simulink model "engine_control_main_sim"  (R2022b)
settings: Solver=VariableStepAuto  StartTime=0.0  StopTime=10.0  RelTol=1e-3
libraries: cstblocks x8
settings Model: Creator=phatdo  LastModifiedBy=phatdo
settings DataIOCC: ReturnWorkspaceOutputs=off

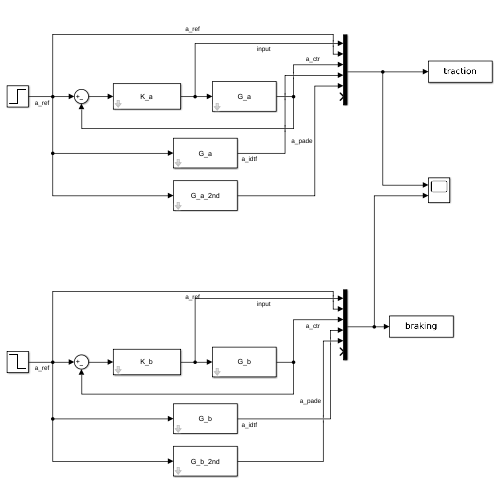
[thumbnail: Simulink's stored preview of the top-level diagram]
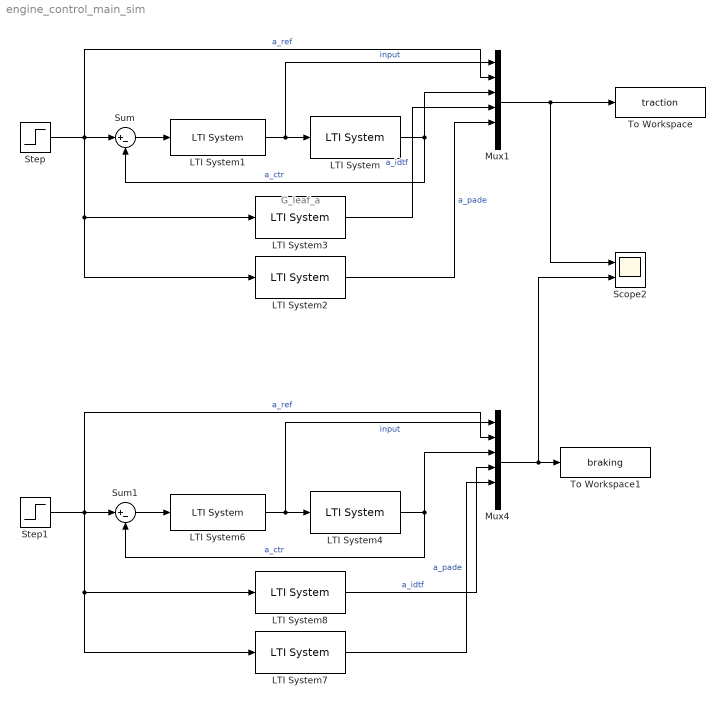
== system engine_control_main_sim ==
  note: G_leaf_a
  LTI System : cstblocks/LTI System  sys=G_a  IC=[]
  LTI System1 : cstblocks/LTI System  sys=K_a  IC=[]
  LTI System2 : cstblocks/LTI System  sys=G_a_2nd  IC=[]
  LTI System3 : cstblocks/LTI System  sys=G_a  IC=[]
  LTI System4 : cstblocks/LTI System  sys=G_b  IC=[]
  LTI System6 : cstblocks/LTI System  sys=K_b  IC=[]
  LTI System7 : cstblocks/LTI System  sys=G_b_2nd  IC=[]
  LTI System8 : cstblocks/LTI System  sys=G_b  IC=[]
  Mux1 : Mux  Inputs=6
  Mux4 : Mux  Inputs=6
  Scope2 : Scope  NumInputPorts=2
  Step : Step  SampleTime=0
  Step1 : Step  After=-1  SampleTime=0
  Sum : Sum  Inputs=|+-
  Sum1 : Sum  Inputs=|+-
  To Workspace : ToWorkspace  VariableName=traction  SaveFormat=Timeseries  SampleTime=-1
  To Workspace1 : ToWorkspace  VariableName=braking  SaveFormat=Timeseries  SampleTime=-1
  wires:
  Step/1 -> Mux1/2, LTI System3/1, LTI System2/1, Sum/1  "a_ref"
  LTI System1/1 -> Mux1/1, LTI System/1  "input"
  Sum/1 -> LTI System1/1
  LTI System/1 -> Mux1/3, Sum/2  "a_ctr"
  LTI System2/1 -> Mux1/5  "a_pade"
  LTI System3/1 -> Mux1/4  "a_idtf"
  LTI System7/1 -> Mux4/5  "a_pade"
  LTI System4/1 -> Mux4/3, Sum1/2  "a_ctr"
  Sum1/1 -> LTI System6/1
  Step1/1 -> Mux4/2, LTI System8/1, LTI System7/1, Sum1/1  "a_ref"
  LTI System8/1 -> Mux4/4  "a_idtf"
  LTI System6/1 -> Mux4/1, LTI System4/1  "input"
  Mux1/1 -> Scope2/1, To Workspace/1
  Mux4/1 -> Scope2/2, To Workspace1/1
